simulink model "practica7comus"  (R2015a)
settings: Solver=FixedStepDiscrete  StartTime=0.0  StopTime=1  FixedStep=0.00001  RelTol=1e-3
libraries: commfilt2 x6, commrandsrc2 x1
settings Model: Creator=hppoc  LastModifiedBy=hppoc

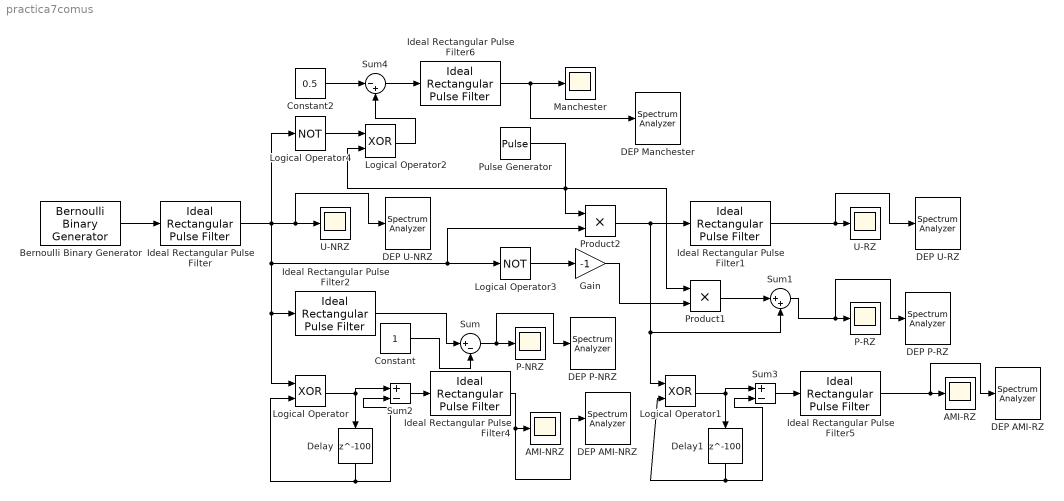
== system practica7comus ==
  AMI-NRZ : Scope
      settings: TimeRange=0.01  YMin=-1.25  YMax=1.25  SaveName=ScopeData4
  AMI-RZ : Scope
      settings: TimeRange=0.01  YMin=-1.25  YMax=1.25  SaveName=ScopeData5
  Bernoulli Binary Generator : commrandsrc2/Bernoulli Binary Generator  P=0.5  seed=randseed  Ts=0.001  frameBased=off  sampPerFrame=1  orient=off  outDataType=int8
  Constant : Constant
  Constant2 : Constant  Value=0.5
  DEP AMI-NRZ : SpectrumAnalyzer
  DEP AMI-RZ : SpectrumAnalyzer
  DEP Manchester : SpectrumAnalyzer
  DEP P-NRZ : SpectrumAnalyzer
  DEP P-RZ : SpectrumAnalyzer
  DEP U-NRZ : SpectrumAnalyzer
  DEP U-RZ : SpectrumAnalyzer
  Delay : Delay  DelayLength=100  InitialCondition=0
  Delay1 : Delay  DelayLength=100  InitialCondition=0
  Gain : Gain  Gain=-1
  Ideal Rectangular Pulse Filter : commfilt2/Ideal Rectangular Pulse Filter  pulseLen=100  pulseDelay=0  sampMode=Allow multirate processing  normCheck=off  normMode=Sum of samples  filterGain=1  roundingMode=Floor  overflowMode=off
  Ideal Rectangular Pulse Filter1 : commfilt2/Ideal Rectangular Pulse Filter  pulseLen=1  pulseDelay=0  sampMode=Enforce single-rate processing  InputProcessing=Columns as channels (frame based)  normCheck=off  normMode=Energy per pulse  filterGain=1  roundingMode=Floor  overflowMode=off  firstCoeffMode=Binary point scaling  firstCoeffWordLength=2  firstCoeffFracLength=0
  Ideal Rectangular Pulse Filter2 : commfilt2/Ideal Rectangular Pulse Filter  pulseLen=1  pulseDelay=0  sampMode=Enforce single-rate processing  InputProcessing=Columns as channels (frame based)  normCheck=off  normMode=Energy per pulse  filterGain=1  roundingMode=Floor  overflowMode=off  firstCoeffMode=Binary point scaling  firstCoeffWordLength=2  firstCoeffFracLength=-1
  Ideal Rectangular Pulse Filter4 : commfilt2/Ideal Rectangular Pulse Filter  pulseLen=1  pulseDelay=0  sampMode=Enforce single-rate processing  InputProcessing=Columns as channels (frame based)  normCheck=off  normMode=Energy per pulse  filterGain=1  roundingMode=Floor  overflowMode=off
  Ideal Rectangular Pulse Filter5 : commfilt2/Ideal Rectangular Pulse Filter  pulseLen=1  pulseDelay=0  sampMode=Enforce single-rate processing  InputProcessing=Columns as channels (frame based)  normCheck=off  normMode=Energy per pulse  filterGain=1  roundingMode=Floor  overflowMode=off
  Ideal Rectangular Pulse Filter6 : commfilt2/Ideal Rectangular Pulse Filter  pulseLen=1  pulseDelay=0  sampMode=Enforce single-rate processing  InputProcessing=Columns as channels (frame based)  normCheck=off  normMode=Energy per pulse  filterGain=2  roundingMode=Floor  overflowMode=off  firstCoeffMode=Binary point scaling  firstCoeffWordLength=2  firstCoeffFracLength=-1
  Logical Operator : Logic  Operator=XOR  AllPortsSameDT=off  OutDataTypeStr=boolean
  Logical Operator1 : Logic  Operator=XOR  AllPortsSameDT=off  OutDataTypeStr=boolean
  Logical Operator2 : Logic  Operator=XOR  AllPortsSameDT=off  OutDataTypeStr=fixdt(1,8)
  Logical Operator3 : Logic  Operator=NOT  AllPortsSameDT=off  OutDataTypeStr=boolean
  Logical Operator4 : Logic  Operator=NOT  AllPortsSameDT=off  OutDataTypeStr=fixdt(1,8)
  Manchester : Scope
      settings: TimeRange=0.01  YMin=-1.25  YMax=1.25  SaveName=ScopeData6
  P-NRZ : Scope
      settings: TimeRange=0.01  YMin=-1.25  YMax=1.25  SaveName=ScopeData2
  P-RZ : Scope
      settings: TimeRange=0.01  YMin=-1.25  YMax=1.25  SaveName=ScopeData3
  Product1 : Product
  Product2 : Product
  Pulse Generator : DiscretePulseGenerator  Period=100  PulseWidth=50  SampleTime=0.00001
  Sum : Sum  Inputs=|+-
  Sum1 : Sum  Inputs=|++
  Sum2 : Sum  Inputs=|+-  OutDataTypeStr=int8
  Sum3 : Sum  Inputs=|+-  AccumDataTypeStr=double  OutDataTypeStr=int8
  Sum4 : Sum  Inputs=|-+
  U-NRZ : Scope
      settings: TimeRange=0.01  YMin=-0.125  YMax=1.125
  U-RZ : Scope
      settings: TimeRange=0.01  YMin=-0.125  YMax=1.125
  wires:
  Ideal Rectangular Pulse Filter1/1 -> DEP U-RZ/1, U-RZ/1
  Ideal Rectangular Pulse Filter2/1 -> Sum/1
  Constant/1 -> Sum/2
  Sum/1 -> P-NRZ/1, DEP P-NRZ/1
  Logical Operator/1 -> Sum2/1, Delay/1
  Delay/1 -> Logical Operator/2, Sum2/2
  Sum2/1 -> Ideal Rectangular Pulse Filter4/1
  Ideal Rectangular Pulse Filter4/1 -> DEP AMI-NRZ/1, AMI-NRZ/1
  Logical Operator1/1 -> Sum3/1, Delay1/1
  Delay1/1 -> Logical Operator1/2, Sum3/2
  Ideal Rectangular Pulse Filter5/1 -> AMI-RZ/1, DEP AMI-RZ/1
  Bernoulli Binary Generator/1 -> Ideal Rectangular Pulse Filter/1
  Sum3/1 -> Ideal Rectangular Pulse Filter5/1
  Ideal Rectangular Pulse Filter/1 -> DEP U-NRZ/1, U-NRZ/1, Logical Operator4/1, Logical Operator/1, Ideal Rectangular Pulse Filter2/1, Product2/2, Logical Operator3/1
  Pulse Generator/1 -> Product2/1, Product1/1, Logical Operator2/2
  Logical Operator4/1 -> Logical Operator2/1
  Ideal Rectangular Pulse Filter6/1 -> Manchester/1, DEP Manchester/1
  Constant2/1 -> Sum4/1
  Sum4/1 -> Ideal Rectangular Pulse Filter6/1
  Logical Operator2/1 -> Sum4/2
  Logical Operator3/1 -> Gain/1
  Gain/1 -> Product1/2
  Product2/1 -> Logical Operator1/1, Sum1/2, Ideal Rectangular Pulse Filter1/1
  Sum1/1 -> DEP P-RZ/1, P-RZ/1
  Product1/1 -> Sum1/1
